simulink model "parallel_battery_SC_boost_converter_new"  (R2021a)
settings: Solver=ode23tb  StartTime=0.0  StopTime=20  RelTol=1e-3  EnableMultiTasking=on
undefined symbols (not defined in the file): Ion, Lithium, Ts
libraries: spsMosfetLib x9, spsSeriesRLCBranchLib x6, spsParallelRLCBranchLib x6, spsVoltageMeasurementLib x5, spsCurrentMeasurementLib x3, slpidlib x3, simulink x3, spsDiodeLib x2, spsThreePhaseParallelRLCLoadLib x1, spsBatteryLib x1, spsIGBTDiodeLib x1, spsThreePhaseVIMeasurementLib x1
settings Model: SimulationMode=accelerator  Creator=The MathWorks, Inc.  LastModifiedBy=JulianChung
settings SolverCC: AlgebraicLoopSolver=TrustRegion
settings DataIOCC: LimitDataPoints=on  SaveFormat=Array  ReturnWorkspaceOutputs=off
settings OptimizationCC: BlockReduction=off  DefaultParameterBehavior=Inlined  BufferReuse=off  ExpressionDepthLimit=2147483647  EfficientMapNaN2IntZero=off  LifeSpan=inf
settings DebuggingCC: UnderspecifiedInitializationDetection=Classic  MergeDetectMultiDrivingBlocksExec=none  SolverPrmCheckMsg=warning  FcnCallInpInsideContextMsg=warning  UnconnectedLineMsg=none  AllowSymbolicDim=off  StateNameClashWarn=warning  SFUnexpectedBacktrackingDiag=warning  SFNoUnconditionalDefaultTransitionDiag=warning  SFExecutionAtInitializationDiag=none  SFMachineParentedDataDiag=warning  ArithmeticOperatorsInVariantConditions=warning
settings HardwareCC: ProdBitPerPointer=32  ProdBitPerSizeT=32  ProdBitPerPtrDiffT=32  ProdLargestAtomicFloat=None  ProdIntDivRoundTo=Undefined  ProdEndianess=Unspecified  ProdWordSize=32  ProdHWDeviceType=32-bit Generic  TargetBitPerPointer=64  TargetBitPerSizeT=64  TargetBitPerPtrDiffT=64  TargetLongLongMode=on  TargetIntDivRoundTo=Zero  TargetEndianess=LittleEndian  TargetWordSize=64  TargetHWDeviceType=MATLAB Host  ProdEqTarget=off
settings ModelReferenceCC: PropagateSignalLabelsOutOfModel=off
settings SFSimCC: SimUseLocalCustomCode=off  CustomCodeUndefinedFunction=UseInterfaceOnly
settings RTWCC: SystemTargetFile=accel.tlc  TemplateMakefile=accel_default_tmf  RTWVerbose=off  RTWUseLocalCustomCode=off
settings CodeAppCC: MaxIdLength=128  StateflowObjectComments=on
settings STFCustomTargetCC: MATLABClassNameForMDSCustomization=Simulink.SoftwareTarget.TargetSpecificTriggerConfigurationBase  UseToolchainInfoCompliant=off  SystemTargetFile=accel.tlc
settings ConfigComp: CovMetricSettings=dw  CovSaveCumulativeToWorkspaceVar=on  CovSaveSingleToWorkspaceVar=on  CovExternalEMLEnable=off  CovSFcnEnable=off
settings SimscapeCC: SimscapeNormalizeSystem=off

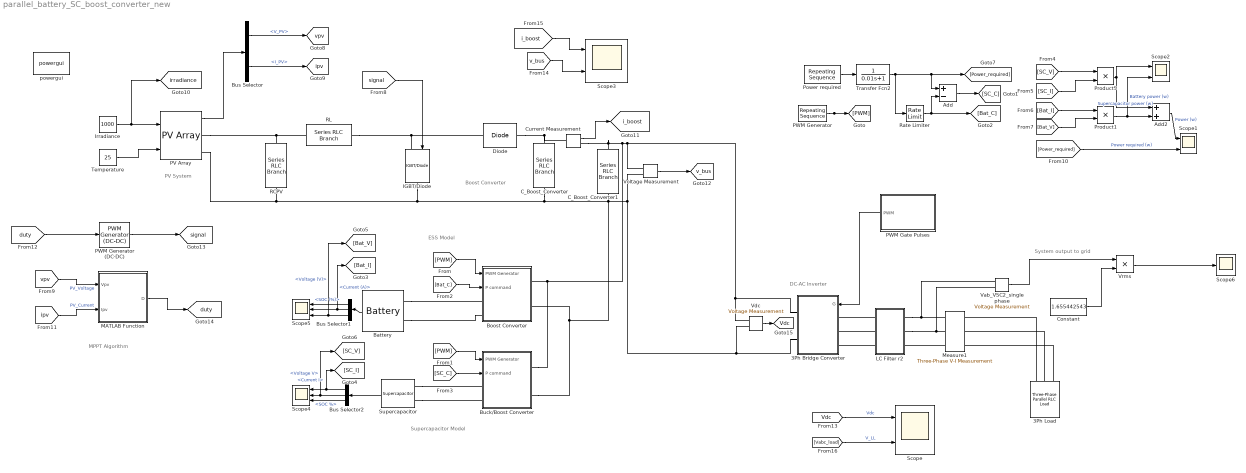
== system parallel_battery_SC_boost_converter_new ==
  note: Supercapacitor Model
  note: MPPT Algorithm
  note: PV System
  note: Boost Converter
  note: DC-AC Inverter
  note: System output to grid
  note: ESS Model
  "3Ph Load " : spsThreePhaseParallelRLCLoadLib/Three-Phase Parallel RLC Load  LConnTagsString=A|B|C  Configuration=Y (floating)  NominalVoltage=415  Vabc=[1e3 1e3 1e3]  Vabcp=[1e3 1e3 1e3]  NominalFrequency=50  UnbalancedPower=off  ActivePower=5e3  InductivePower=0  CapacitivePower=0  Pabc=[10e3 9e3 11e3]  QLabc=[100 90 110]  QCabc=[100 90 110]  Pabcp=[10e3 9e3 11e3]  QLabcp=[100 90 110]  QCabcp=[100 90 110]  Measurements=None  LoadType=constant Z
  3Ph Bridge Converter : Subsystem
  Add : Sum  Inputs=+-
  Add2 : Sum
  Battery : spsBatteryLib/Battery  BatType=Lithium-Ion  ShowTempParam=off  ThermalPreset=no  ShowAgeParam=off  NomV=26.4  NomQ=6.6  SOC=100  Batt_Tr=30  PresetModel=on  MaxQ=6.6  MinV=19.8  FullV=30.7293  Dis_rate=2.8696  R=0.04  Normal_OP=5.9687  expZone="[28.5222     0.324261]"  current=[6.5 13 32.5]  Units=Time  Tci=20  NomT=25  T2=0  MaxQ2=2.208  FullV2=3.45  Normal_OP2=2.8  expZone2="[3.22        0.23]"  Rca=0.6  ti=1000  Dp=0  Neq0=0  Tsim=1e6  Ta1=25  Qeol=5.4*0.9  Reol=0.013333*1.2  Char_age=[2.3478, 3]  Dis_age=[2.3478, 10]  N1=1500  N2=10500  N3=1000  N4=1400  Ta2=45  N5=950
  Boost Converter : Subsystem
  Buck/Boost Converter : Subsystem
  Bus Selector : BusSelector  OutputSignals=V_PV,I_PV
  Bus Selector1 : BusSelector  OutputSignals=SOC (%),Current (A),Voltage (V)
  Bus Selector2 : BusSelector  OutputSignals=Current I,Voltage V,SOC %
  C_Boost_Converter : spsSeriesRLCBranchLib/Series RLC Branch  LConnTagsString=__new0  RConnTagsString=__new0  BranchType=RC  Resistance=1e-4  Inductance=1e-3  SetiL0=off  InitialCurrent=0  Capacitance=3300e-6  Setx0=off  InitialVoltage=0  Measurements=None
  C_Boost_Converter1 : spsSeriesRLCBranchLib/Series RLC Branch  LConnTagsString=__new0  RConnTagsString=__new0  BranchType=R  Resistance=12  Inductance=1e-3  SetiL0=off  InitialCurrent=0  Capacitance=3300e-6  Setx0=off  InitialVoltage=0  Measurements=None
  Constant : Constant  Value=1.655442543
  Current Measurement : spsCurrentMeasurementLib/Current Measurement  PhasorSimulation=off  OutputType=Complex  PSBequivalent=0
  Diode : spsDiodeLib/Diode  Ron=0.001  Lon=0  Vf=0.8  IC=0  UseSnubber=0  Rs=500  Cs=250e-9  Measurements=off
  IGBT/Diode : spsIGBTDiodeLib/IGBT//Diode  Ron=1e-3  Rs=1e5  Cs=inf  Measurements=off
  Irradiance : Constant  Value=1000
  LC Filter r2 : Subsystem  mask{L=10e-3, C=20e-6}
      mask prompts: L "Inductance"; C "Capacitance"
  MATLAB Function : MATLAB Function  TreatAsAtomicUnit=on
  Measure1 : spsThreePhaseVIMeasurementLib/Three-Phase V-I Measurement  VoltageMeasurement=phase-to-phase  SetLabelV=on  LabelV=Vabc_load  Vpu=off  VpuLL=off  CurrentMeasurement=no  SetLabelI=off  LabelI=I1  Ipu=off  Pbase=1e3  Vbase=380  OutputType=Magnitude  PhasorSimulation=off  PSBequivalent=0
  PV Array : spsPVArrayLib/PV Array  Npar=10  Nser=3  PlotType=array @ 1000 W/m2 & specified temperatures  S_vec="[ 1000  500  100 ]"  Temp_C_vec="[ 45 25  ]"  ModuleName=User-defined  PlotWhenSelected=off  Pm=30  Ncell=20  Voc=12  Isc=4  Vm=10  Im=3  beta_Voc_pc=-0.318  alpha_Isc_pc=0.011  beta_Voc=-0.03816  alpha_Isc=0.00044  IL=4.052  I0=2.3913e-11  nI=0.9143  Rsh=11.0082  Rs=0.14305  RobustModel=off  RobustCellTemperature=313.3991  BAL=on  Tc=1e-6  Tfilter=5e-5
  PWM Gate Pulses : Subsystem  mask{fc=50, fs=20000, m=1, inj=off, shift=0}
      mask prompts: fc "Control signal freq(Fc)"; fs "Swicting frequency"; m "Modulation Index"; inj "3rd harmonic Injection"; shift "Phase shift(Degrees)"
  PWM Generator : simulink/Sources/Repeating Sequence  rep_seq_t="[0 1/4*0.0001  2/4*0.0001  3/4*0.0001  0.0001]"  rep_seq_y=[0 1 0 -1 0]
  PWM Generator (DC-DC) : spsPWMGeneratorDCDCLib/PWM Generator (DC-DC)  Fsw=5000  Ts=10e-6
  Power required : simulink/Sources/Repeating Sequence  rep_seq_t=[0 1 2 3 5 6 7 8 9 10]  rep_seq_y=[2000 1500 1250 1000 1000 1000 500 0 0 0 ]
  Product1 : Product  RndMeth=Zero
  Product5 : Product  RndMeth=Zero
  RCPV : spsSeriesRLCBranchLib/Series RLC Branch  LConnTagsString=__new0  RConnTagsString=__new0  BranchType=RC  Resistance=1e-4  Inductance=1e-3  SetiL0=off  InitialCurrent=0  Capacitance=100e-6  Setx0=off  InitialVoltage=0  Measurements=None
  RL : spsSeriesRLCBranchLib/Series RLC Branch  LConnTagsString=__new0  RConnTagsString=__new0  BranchType=RL  Resistance=0.1  Inductance=5e-3  SetiL0=off  InitialCurrent=0  Capacitance=100e-6  Setx0=off  InitialVoltage=0  Measurements=None
  Rate Limiter : RateLimiter  RisingSlewLimit=300  FallingSlewLimit=-300  SampleTimeMode=inherited
  Scope{,1..3} (4 alike) : Scope  NumInputPorts=2
  Scope4 : Scope  NumInputPorts=3
  Scope5 : Scope  NumInputPorts=3
  Scope6 : Scope
  Supercapacitor : spsSupercapacitorLib/Supercapacitor  C=500  Rdc=2.1e-3  Voltage=16  Ns=6  Np=1  Vinit=16  Temp=25  PresetModel=on  EstParam=off  Nc=1  r=1e-9  epsilon=6.0208e-10  Ich=10  Vstern="[0.161  2.7  7.8]"  Self_dis=on  Ioc=10  Vself="[48  47.8  47.06  44.65]"  demandeplot=off  I=10.2  Units=sec  Vmax=17  If=5.2e-3  deltaV=0.3  alpha=0.3  sec=1988
      settings: SourceProductBaseCode=PS
  Temperature : Constant  Value=25
  Transfer Fcn2 : TransferFcn  Denominator=[0.01 1]
  Vab_VSC2_single phase : spsVoltageMeasurementLib/Voltage Measurement  Tag=PoWeRsYsTeMmEaSuReMeNt  PhasorSimulation=off  OutputType=Magnitude  PSBequivalent=0
  "Vdc " : spsVoltageMeasurementLib/Voltage Measurement  Tag=PoWeRsYsTeMmEaSuReMeNt  PhasorSimulation=off  OutputType=Magnitude  PSBequivalent=0
  Voltage Measurement : spsVoltageMeasurementLib/Voltage Measurement  PhasorSimulation=off  OutputType=Complex  PSBequivalent=0
  Vrms : Product
  powergui : spspowerguiLib/powergui  Priority=1  SimulationMode=Discrete  SampleTime=10e-6  frequency=60  Iterations=50  frequencyindice=0  Pbase=100e6  ErrMax=1e-4  UnitsV=kV  UnitsW=MW  buscounter=0  FunctionMessages=off  echomessages=off  EnableUseOfTLC=off  CurrentSourceSwitches=off  DisableSnubberDevices=off  DisableRonSwitches=off  DisableVfSwitches=off  DisplayEquations=off  AutomaticDiscreteSolvers=off  SolverType=Tustin/Backward Euler (TBE)  Interpol=off  ExternalGateDelay=off  methode=off  Ts=0  x0status=blocks  SPID=off  SwTol=0  HookPort=off  NonlinearTolerance=1e-4  nMaxIteration=100  ContinueOnMaxIteration=off  RestoreLinks=warning  ResistiveCurrentMeasurement=off  Frange=[0:1:1000]  Ylog=on  Xlog=on  ShowGrid=on  save=on  variable=ZDa  structure=donnee  ZoomFFT=off  StartTime=0.0  cycles=1  DisplayStyle=1  fundamental=60  FreqAxis=off  MaxFrequency=1000  frequencyindicesteady=10  RmsSteady=1  display=off
  tag scope: Vdc=global, duty=global, i_boost=global, ipv=global, irradiance=global, signal=global, v_bus=global, vpv=global
  wires:
  Battery/1 -> Bus Selector1/1
  Bus Selector1/1 -> Scope5/1  "<SOC (%)>"
  Bus Selector1/2 -> [Bat_I], Scope5/2  "<Current (A)>"
  Bus Selector1/3 -> Scope5/3, [Bat_V]  "<Voltage (V)>"
  Transfer Fcn2/1 -> Rate Limiter/1, Add/1, [Power_required]
  Rate Limiter/1 -> Add/2, [Bat_C]
  Power required/1 -> Transfer Fcn2/1
  PWM Generator/1 -> [PWM]
  [PWM] -> Boost Converter/1(PWM Generator)
  [Bat_C] -> Boost Converter/2(P command)
  [PWM] -> Buck/Boost Converter/1(PWM Generator)
  [SC_C] -> Buck/Boost Converter/2(P command)
  Add/1 -> [SC_C]
  Bus Selector2/1 -> [SC_I], Scope4/1  "<Current I>"
  Bus Selector2/2 -> Scope4/2, [SC_V]  "<Voltage V>"
  Bus Selector2/3 -> Scope4/3  "<SOC %>"
  Supercapacitor/1 -> Bus Selector2/1
  [Bat_I] -> Product1/1
  [Bat_V] -> Product1/2
  [SC_V] -> Product5/1
  [SC_I] -> Product5/2
  Product5/1 -> Add2/1, Scope2/1  "Supercapacitor power (w)"
  Product1/1 -> Add2/2, Scope2/2  "Battery power (w)"
  [Power_required] -> Scope1/2  "Power required (w)"
  Add2/1 -> Scope1/1  "Power (w)"
  Bus Selector/1 -> [vpv]  "<V_PV>"
  Voltage Measurement/1 -> [v_bus]
  Current Measurement/1 -> [i_boost]
  [signal] -> IGBT/Diode/1
  PV Array/1 -> Bus Selector/1
  Bus Selector/2 -> [ipv]  "<I_PV>"
  Irradiance/1 -> [irradiance], PV Array/1
  Temperature/1 -> PV Array/2
  [ipv] -> MATLAB Function/2(Ipv)  "PV_Current"
  [vpv] -> MATLAB Function/1(Vpv)  "PV_Voltage"
  MATLAB Function/1(D) -> [duty]
  PWM Generator (DC-DC)/1 -> [signal]
  [duty] -> PWM Generator (DC-DC)/1
  [i_boost] -> Scope3/1
  [v_bus] -> Scope3/2
  PWM Gate Pulses/1(PWM) -> 3Ph Bridge Converter/1(G)
  "Vdc "/1 -> [Vdc]
  [Vdc] -> Scope/1  "Vdc"
  [Vabc_load] -> Scope/2  "V_LL"
  Vab_VSC2_single phase/1 -> Vrms/1
  Constant/1 -> Vrms/2
  Vrms/1 -> Scope6/1
  connections:
  Supercapacitor/LConn1 -- Buck/Boost Converter/LConn1
  Supercapacitor/LConn2 -- Buck/Boost Converter/LConn2
  Battery/LConn1 -- Boost Converter/LConn1
  Battery/LConn2 -- Boost Converter/LConn2
  3Ph Bridge Converter/RConn2 -- "Vdc "/LConn2 -- Voltage Measurement/LConn2 -- Boost Converter/RConn2 -- Buck/Boost Converter/RConn2 -- C_Boost_Converter1/RConn1 -- RCPV/RConn1 -- PV Array/RConn2 -- IGBT/Diode/RConn1 -- C_Boost_Converter/RConn1
  Diode/LConn1 -- RL/LConn1 -- IGBT/Diode/LConn1
  3Ph Bridge Converter/RConn1 -- C_Boost_Converter1/LConn1 -- Current Measurement/RConn1 -- Boost Converter/RConn1 -- Buck/Boost Converter/RConn1 -- Voltage Measurement/LConn1 -- "Vdc "/LConn1
  RCPV/LConn1 -- RL/RConn1 -- PV Array/RConn1
  Diode/RConn1 -- C_Boost_Converter/LConn1 -- Current Measurement/LConn1
  Measure1/LConn2 -- Vab_VSC2_single phase/LConn2 -- LC Filter r2/RConn2
  LC Filter r2/RConn1 -- Vab_VSC2_single phase/LConn1 -- Measure1/LConn1
  Measure1/LConn3 -- LC Filter r2/RConn3
  "3Ph Load "/LConn1 -- Measure1/RConn1
  LC Filter r2/LConn2 -- 3Ph Bridge Converter/LConn2
  "3Ph Load "/LConn2 -- Measure1/RConn2
  LC Filter r2/LConn3 -- 3Ph Bridge Converter/LConn3
  LC Filter r2/LConn1 -- 3Ph Bridge Converter/LConn1
  "3Ph Load "/LConn3 -- Measure1/RConn3

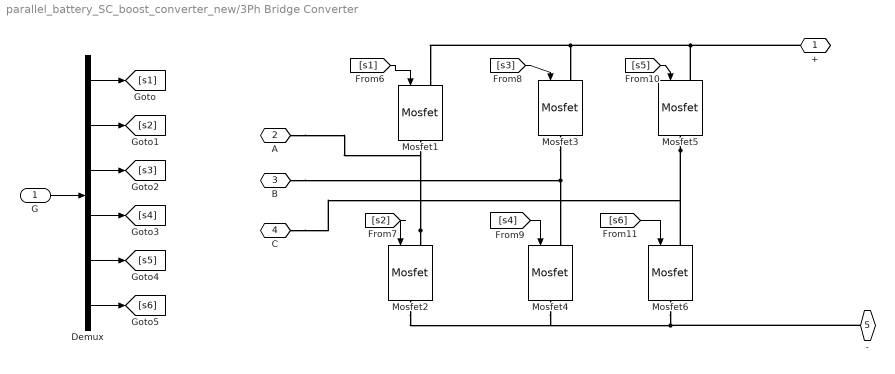
== system parallel_battery_SC_boost_converter_new/3Ph Bridge Converter ==
  G : Inport
  Demux : Demux  Outputs=6
  Mosfet{1..6} (6 alike) : spsMosfetLib/Mosfet  Ron=0.1  Lon=0  Rd=0.01  Vfd=0  IC=0  Rs=1e5  Cs=inf  Measurements=off
  + : PMIOPort  Side=Right
  A : PMIOPort  Port=2  Side=Left
  B : PMIOPort  Port=3  Side=Left
  C : PMIOPort  Port=4  Side=Left
  - : PMIOPort  Port=5  Side=Right
  wires:
  [s1] -> Mosfet1/1
  [s2] -> Mosfet2/1
  [s3] -> Mosfet3/1
  [s4] -> Mosfet4/1
  [s5] -> Mosfet5/1
  [s6] -> Mosfet6/1
  Demux/1 -> [s1]
  Demux/2 -> [s2]
  Demux/3 -> [s3]
  Demux/4 -> [s4]
  Demux/5 -> [s5]
  Demux/6 -> [s6]
  G/1 -> Demux/1
  connections:
  Mosfet5/LConn1 -- Mosfet1/LConn1 -- Mosfet3/LConn1 -- +/RConn1
  Mosfet6/RConn1 -- Mosfet2/RConn1 -- Mosfet4/RConn1 -- -/RConn1
  Mosfet2/LConn1 -- Mosfet1/RConn1 -- A/RConn1
  Mosfet3/RConn1 -- Mosfet4/LConn1 -- B/RConn1
  Mosfet5/RConn1 -- Mosfet6/LConn1 -- C/RConn1

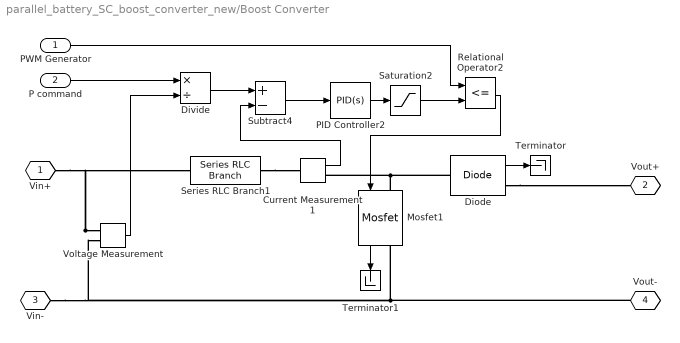
== system parallel_battery_SC_boost_converter_new/Boost Converter ==
  PWM Generator : Inport
  P command : Inport  Port=2
  Current Measurement1 : spsCurrentMeasurementLib/Current Measurement  PhasorSimulation=off  OutputType=Complex  PSBequivalent=0
  Diode : spsDiodeLib/Diode  Ron=0.001  Lon=0  Vf=0.8  IC=0  UseSnubber=off  Rs=500  Cs=250e-9  Measurements=on
  Divide : Product  Inputs=*/
  Mosfet1 : spsMosfetLib/Mosfet  Ron=0.1  Lon=0  Rd=0.01  Vfd=0  IC=0  Rs=1e5  Cs=inf  Measurements=on
  PID Controller2 : slpidlib/PID Controller  Controller=PID  Form=Parallel  TimeDomain=Continuous-time  UseExternalTs=off  SampleTime=-1  IntegratorMethod=Forward Euler  FilterMethod=Forward Euler  ControllerParametersSource=internal  P=1.5  I=1  D=0  UseFilter=on  N=100  TunerSelectOption=Transfer Function Based (PID Tuner App)  InitialConditionSource=internal  InitialConditionForIntegrator=0  InitialConditionForFilter=0  DifferentiatorICPrevScaledInput=0  ExternalReset=none  TrackingMode=off  Kt=1  LimitOutput=off  SatLimitsSource=internal  UpperSaturationLimit=inf  LowerSaturationLimit=-inf  LinearizeAsGain=off  AntiWindupMode=none  Kb=1  POutMin=[]  POutMax=[]  IOutMin=[]  IOutMax=[]  DOutMin=[]  DOutMax=[]  NOutMin=[]  NOutMax=[]  SumOutMin=[]  SumOutMax=[]  SaturationOutMin=[]  SaturationOutMax=[]  PParamMin=[]  PParamMax=[]  IParamMin=[]  IParamMax=[]  DParamMin=[]  DParamMax=[]  NParamMin=[]  NParamMax=[]  KbParamMin=[]  KbParamMax=[]  KtParamMin=[]  KtParamMax=[]  KbOutMin=[]  KbOutMax=[]  KtOutMin=[]  KtOutMax=[]  IntegratorOutMin=[]  IntegratorOutMax=[]  FilterOutMin=[]  FilterOutMax=[]  SumI1OutMin=[]  SumI1OutMax=[]  SumI2OutMin=[]  SumI2OutMax=[]  SumI3OutMin=[]  SumI3OutMax=[]  SumI4OutMin=[]  SumI4OutMax=[]  SumDOutMin=[]  SumDOutMax=[]  DifferentiatorOutMin=[]  DifferentiatorOutMax=[]  FilterDiffOutCoefMin=[]  FilterDiffOutCoefMax=[]  ReciprocalOutMin=[]  ReciprocalOutMax=[]  SumDenOutMin=[]  SumDenOutMax=[]  SumNumOutMin=[]  SumNumOutMax=[]  DivideOutMin=[]  DivideOutMax=[]  UdiffTsProdOutMin=[]  UdiffTsProdOutMax=[]  NTsProdOutMin=[]  NTsProdOutMax=[]  UintegralTsProdOutMin=[]  UintegralTsProdOutMax=[]  UngainTsProdOutMin=[]  UngainTsProdOutMax=[]  IntegratorContinuousStateAttributes=''  IntegratorStateMustResolveToSignalObject=off  IntegratorRTWStateStorageClass=Auto  FilterContinuousStateAttributes=''  FilterStateMustResolveToSignalObject=off  FilterRTWStateStorageClass=Auto  ParallelPVariant=InternalParameters  IdealPVariant=Disabled  IVariant=InternalParameters  DVariant=InternalParameters  IntegratorVariant=Continuous  SatVariant=Disabled  AWVariant=Passthrough  PCopyVariant=Disabled  TRVariant=Disabled  FdbkBlocksVariant=Forward  IdealPFdbkVariant=Disabled  SatFdbkVariant=Disabled  DerivativeFilterVariant=ContFilter  NVariant=InternalParameters  NCopyVariant=Disabled  FilterICVariant=InternalICsFilter  IntegratorICVariant=InternalICs  ExternalResetVariant=Disabled  TRSumVariant=Passthrough  SumFdbkVariant=Disabled  SumVariant=Sum_PID  TsampFilterVariant=InternalTs  TsampNgainVariant=Passthrough  TsampIntegralVariant=Passthrough  ExternalSaturationOutDataTypeStr=Inherit: Same as second input
  Relational Operator2 : RelationalOperator  Operator=<=  OutDataTypeStr=boolean  RndMeth=Nearest
  Saturation2 : Saturate  UpperLimit=1  LowerLimit=-1
  Series RLC Branch1 : spsSeriesRLCBranchLib/Series RLC Branch  LConnTagsString=__new0  RConnTagsString=__new0  BranchType=L  Resistance=1  Inductance=1e-3  SetiL0=off  InitialCurrent=0  Capacitance=1e-6  Setx0=off  InitialVoltage=0  Measurements=None
  Subtract4 : Sum  Inputs=+-
  Terminator : Terminator
  Terminator1 : Terminator
  Voltage Measurement : spsVoltageMeasurementLib/Voltage Measurement  PhasorSimulation=off  OutputType=Complex  PSBequivalent=0
  Vin+ : PMIOPort  Tag=PMCPort  Side=Left
  Vout+ : PMIOPort  Tag=PMCPort  Port=2  Side=Right
  Vin- : PMIOPort  Tag=PMCPort  Port=3  Side=Left
  Vout- : PMIOPort  Tag=PMCPort  Port=4  Side=Right
  wires:
  Voltage Measurement/1 -> Divide/2
  P command/1 -> Divide/1
  Divide/1 -> Subtract4/1
  Relational Operator2/1 -> Mosfet1/1
  Current Measurement1/1 -> Subtract4/2
  PWM Generator/1 -> Relational Operator2/1
  Subtract4/1 -> PID Controller2/1
  PID Controller2/1 -> Saturation2/1
  Saturation2/1 -> Relational Operator2/2
  Diode/1 -> Terminator/1
  Mosfet1/1 -> Terminator1/1
  connections:
  Series RLC Branch1/RConn1 -- Current Measurement1/LConn1
  Vout-/RConn1 -- Voltage Measurement/LConn2 -- Vin-/RConn1 -- Mosfet1/RConn1
  Voltage Measurement/LConn1 -- Series RLC Branch1/LConn1 -- Vin+/RConn1
  Diode/LConn1 -- Current Measurement1/RConn1 -- Mosfet1/LConn1
  Diode/RConn1 -- Vout+/RConn1

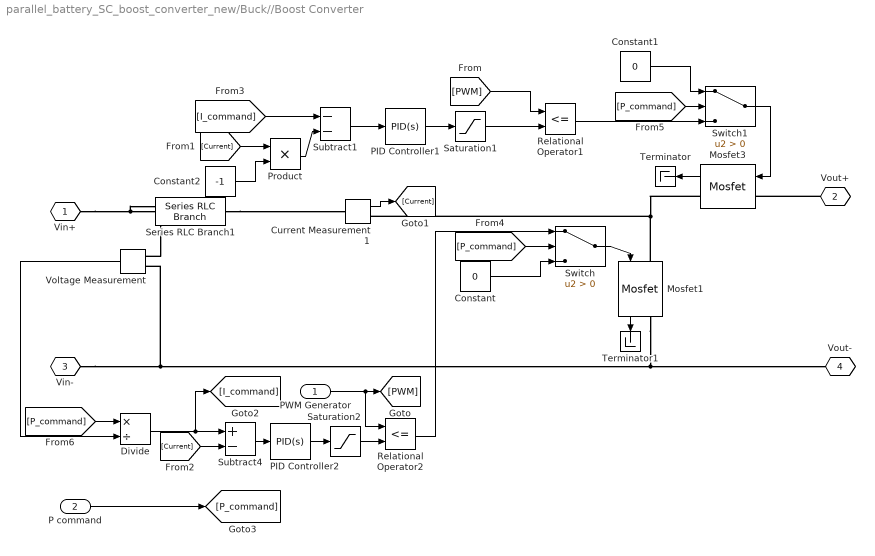
== system parallel_battery_SC_boost_converter_new/Buck//Boost Converter ==
  PWM Generator : Inport
  P command : Inport  Port=2
  Constant : Constant  Value=0
  Constant1 : Constant  Value=0
  Constant2 : Constant  Value=-1
  Current Measurement1 : spsCurrentMeasurementLib/Current Measurement  PhasorSimulation=off  OutputType=Complex  PSBequivalent=0
  Divide : Product  Inputs=*/
  Mosfet1 : spsMosfetLib/Mosfet  Ron=0.1  Lon=0  Rd=0.01  Vfd=0  IC=0  Rs=1e5  Cs=inf  Measurements=on
  Mosfet3 : spsMosfetLib/Mosfet  Ron=0.1  Lon=0  Rd=0.01  Vfd=0  IC=0  Rs=1e5  Cs=inf  Measurements=on
  PID Controller1 : slpidlib/PID Controller  Controller=PID  Form=Parallel  TimeDomain=Continuous-time  UseExternalTs=off  SampleTime=-1  IntegratorMethod=Forward Euler  FilterMethod=Forward Euler  ControllerParametersSource=internal  P=1.5  I=1  D=0  UseFilter=on  N=100  TunerSelectOption=Transfer Function Based (PID Tuner App)  InitialConditionSource=internal  InitialConditionForIntegrator=0  InitialConditionForFilter=0  DifferentiatorICPrevScaledInput=0  ExternalReset=none  TrackingMode=off  Kt=1  LimitOutput=off  SatLimitsSource=internal  UpperSaturationLimit=inf  LowerSaturationLimit=-inf  LinearizeAsGain=off  AntiWindupMode=none  Kb=1  POutMin=[]  POutMax=[]  IOutMin=[]  IOutMax=[]  DOutMin=[]  DOutMax=[]  NOutMin=[]  NOutMax=[]  SumOutMin=[]  SumOutMax=[]  SaturationOutMin=[]  SaturationOutMax=[]  PParamMin=[]  PParamMax=[]  IParamMin=[]  IParamMax=[]  DParamMin=[]  DParamMax=[]  NParamMin=[]  NParamMax=[]  KbParamMin=[]  KbParamMax=[]  KtParamMin=[]  KtParamMax=[]  KbOutMin=[]  KbOutMax=[]  KtOutMin=[]  KtOutMax=[]  IntegratorOutMin=[]  IntegratorOutMax=[]  FilterOutMin=[]  FilterOutMax=[]  SumI1OutMin=[]  SumI1OutMax=[]  SumI2OutMin=[]  SumI2OutMax=[]  SumI3OutMin=[]  SumI3OutMax=[]  SumI4OutMin=[]  SumI4OutMax=[]  SumDOutMin=[]  SumDOutMax=[]  DifferentiatorOutMin=[]  DifferentiatorOutMax=[]  FilterDiffOutCoefMin=[]  FilterDiffOutCoefMax=[]  ReciprocalOutMin=[]  ReciprocalOutMax=[]  SumDenOutMin=[]  SumDenOutMax=[]  SumNumOutMin=[]  SumNumOutMax=[]  DivideOutMin=[]  DivideOutMax=[]  UdiffTsProdOutMin=[]  UdiffTsProdOutMax=[]  NTsProdOutMin=[]  NTsProdOutMax=[]  UintegralTsProdOutMin=[]  UintegralTsProdOutMax=[]  UngainTsProdOutMin=[]  UngainTsProdOutMax=[]  IntegratorContinuousStateAttributes=''  IntegratorStateMustResolveToSignalObject=off  IntegratorRTWStateStorageClass=Auto  FilterContinuousStateAttributes=''  FilterStateMustResolveToSignalObject=off  FilterRTWStateStorageClass=Auto  ParallelPVariant=InternalParameters  IdealPVariant=Disabled  IVariant=InternalParameters  DVariant=InternalParameters  IntegratorVariant=Continuous  SatVariant=Disabled  AWVariant=Passthrough  PCopyVariant=Disabled  TRVariant=Disabled  FdbkBlocksVariant=Forward  IdealPFdbkVariant=Disabled  SatFdbkVariant=Disabled  DerivativeFilterVariant=ContFilter  NVariant=InternalParameters  NCopyVariant=Disabled  FilterICVariant=InternalICsFilter  IntegratorICVariant=InternalICs  ExternalResetVariant=Disabled  TRSumVariant=Passthrough  SumFdbkVariant=Disabled  SumVariant=Sum_PID  TsampFilterVariant=InternalTs  TsampNgainVariant=Passthrough  TsampIntegralVariant=Passthrough  ExternalSaturationOutDataTypeStr=Inherit: Same as second input
  PID Controller2 : slpidlib/PID Controller  Controller=PID  Form=Parallel  TimeDomain=Continuous-time  UseExternalTs=off  SampleTime=-1  IntegratorMethod=Forward Euler  FilterMethod=Forward Euler  ControllerParametersSource=internal  P=1.5  I=1  D=0  UseFilter=on  N=100  TunerSelectOption=Transfer Function Based (PID Tuner App)  InitialConditionSource=internal  InitialConditionForIntegrator=0  InitialConditionForFilter=0  DifferentiatorICPrevScaledInput=0  ExternalReset=none  TrackingMode=off  Kt=1  LimitOutput=off  SatLimitsSource=internal  UpperSaturationLimit=inf  LowerSaturationLimit=-inf  LinearizeAsGain=off  AntiWindupMode=none  Kb=1  POutMin=[]  POutMax=[]  IOutMin=[]  IOutMax=[]  DOutMin=[]  DOutMax=[]  NOutMin=[]  NOutMax=[]  SumOutMin=[]  SumOutMax=[]  SaturationOutMin=[]  SaturationOutMax=[]  PParamMin=[]  PParamMax=[]  IParamMin=[]  IParamMax=[]  DParamMin=[]  DParamMax=[]  NParamMin=[]  NParamMax=[]  KbParamMin=[]  KbParamMax=[]  KtParamMin=[]  KtParamMax=[]  KbOutMin=[]  KbOutMax=[]  KtOutMin=[]  KtOutMax=[]  IntegratorOutMin=[]  IntegratorOutMax=[]  FilterOutMin=[]  FilterOutMax=[]  SumI1OutMin=[]  SumI1OutMax=[]  SumI2OutMin=[]  SumI2OutMax=[]  SumI3OutMin=[]  SumI3OutMax=[]  SumI4OutMin=[]  SumI4OutMax=[]  SumDOutMin=[]  SumDOutMax=[]  DifferentiatorOutMin=[]  DifferentiatorOutMax=[]  FilterDiffOutCoefMin=[]  FilterDiffOutCoefMax=[]  ReciprocalOutMin=[]  ReciprocalOutMax=[]  SumDenOutMin=[]  SumDenOutMax=[]  SumNumOutMin=[]  SumNumOutMax=[]  DivideOutMin=[]  DivideOutMax=[]  UdiffTsProdOutMin=[]  UdiffTsProdOutMax=[]  NTsProdOutMin=[]  NTsProdOutMax=[]  UintegralTsProdOutMin=[]  UintegralTsProdOutMax=[]  UngainTsProdOutMin=[]  UngainTsProdOutMax=[]  IntegratorContinuousStateAttributes=''  IntegratorStateMustResolveToSignalObject=off  IntegratorRTWStateStorageClass=Auto  FilterContinuousStateAttributes=''  FilterStateMustResolveToSignalObject=off  FilterRTWStateStorageClass=Auto  ParallelPVariant=InternalParameters  IdealPVariant=Disabled  IVariant=InternalParameters  DVariant=InternalParameters  IntegratorVariant=Continuous  SatVariant=Disabled  AWVariant=Passthrough  PCopyVariant=Disabled  TRVariant=Disabled  FdbkBlocksVariant=Forward  IdealPFdbkVariant=Disabled  SatFdbkVariant=Disabled  DerivativeFilterVariant=ContFilter  NVariant=InternalParameters  NCopyVariant=Disabled  FilterICVariant=InternalICsFilter  IntegratorICVariant=InternalICs  ExternalResetVariant=Disabled  TRSumVariant=Passthrough  SumFdbkVariant=Disabled  SumVariant=Sum_PID  TsampFilterVariant=InternalTs  TsampNgainVariant=Passthrough  TsampIntegralVariant=Passthrough  ExternalSaturationOutDataTypeStr=Inherit: Same as second input
  Product : Product  RndMeth=Zero
  Relational Operator1 : RelationalOperator  Operator=<=  OutDataTypeStr=boolean  RndMeth=Nearest
  Relational Operator2 : RelationalOperator  Operator=<=  OutDataTypeStr=boolean  RndMeth=Nearest
  Saturation1 : Saturate  UpperLimit=1  LowerLimit=-1
  Saturation2 : Saturate  UpperLimit=1  LowerLimit=-1
  Series RLC Branch1 : spsSeriesRLCBranchLib/Series RLC Branch  LConnTagsString=__new0  RConnTagsString=__new0  BranchType=L  Resistance=1  Inductance=1e-3  SetiL0=off  InitialCurrent=0  Capacitance=1e-6  Setx0=off  InitialVoltage=0  Measurements=None
  Subtract1 : Sum  Inputs=--
  Subtract4 : Sum  Inputs=+-
  Switch : Switch  Criteria=u2 > Threshold
  Switch1 : Switch  Criteria=u2 > Threshold
  Terminator : Terminator
  Terminator1 : Terminator
  Voltage Measurement : spsVoltageMeasurementLib/Voltage Measurement  PhasorSimulation=off  OutputType=Complex  PSBequivalent=0
  Vin+ : PMIOPort  Tag=PMCPort  Side=Left
  Vout+ : PMIOPort  Tag=PMCPort  Port=2  Side=Right
  Vin- : PMIOPort  Tag=PMCPort  Port=3  Side=Left
  Vout- : PMIOPort  Tag=PMCPort  Port=4  Side=Right
  wires:
  Saturation2/1 -> Relational Operator2/2
  PID Controller2/1 -> Saturation2/1
  Subtract4/1 -> PID Controller2/1
  PWM Generator/1 -> Relational Operator2/1, [PWM]
  Divide/1 -> [I_command], Subtract4/1
  P command/1 -> [P_command]
  Switch/1 -> Mosfet1/1
  Saturation1/1 -> Relational Operator1/2
  PID Controller1/1 -> Saturation1/1
  Subtract1/1 -> PID Controller1/1
  [PWM] -> Relational Operator1/1
  [Current] -> Subtract4/2
  [Current] -> Product/1
  Product/1 -> Subtract1/2
  Constant2/1 -> Product/2
  [I_command] -> Subtract1/1
  Current Measurement1/1 -> [Current]
  Switch1/1 -> Mosfet3/1
  Relational Operator2/1 -> Switch/1
  Constant/1 -> Switch/3
  Constant1/1 -> Switch1/1
  Mosfet3/1 -> Terminator/1
  Mosfet1/1 -> Terminator1/1
  Relational Operator1/1 -> Switch1/3
  [P_command] -> Switch/2
  [P_command] -> Switch1/2
  [P_command] -> Divide/1
  Voltage Measurement/1 -> Divide/2
  connections:
  Vin-/RConn1 -- Voltage Measurement/LConn2 -- Vout-/RConn1 -- Mosfet1/RConn1
  Vin+/RConn1 -- Series RLC Branch1/LConn1 -- Voltage Measurement/LConn1
  Mosfet1/LConn1 -- Current Measurement1/RConn1 -- Mosfet3/RConn1
  Series RLC Branch1/RConn1 -- Current Measurement1/LConn1
  Vout+/RConn1 -- Mosfet3/LConn1

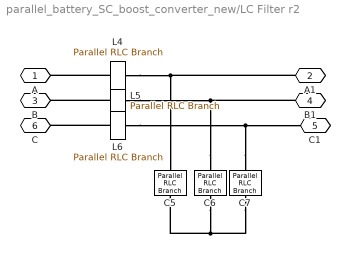
== system parallel_battery_SC_boost_converter_new/LC Filter r2 ==
  C5 : spsParallelRLCBranchLib/Parallel RLC Branch  LConnTagsString=a  RConnTagsString=__new0  BranchType=C  Resistance=inf  Inductance=inf  SetiL0=off  InitialCurrent=0  Capacitance=C  Setx0=off  InitialVoltage=0  Measurements=None
  C6 : spsParallelRLCBranchLib/Parallel RLC Branch  LConnTagsString=a  RConnTagsString=__new0  BranchType=C  Resistance=inf  Inductance=inf  SetiL0=off  InitialCurrent=0  Capacitance=C  Setx0=off  InitialVoltage=0  Measurements=None
  C7 : spsParallelRLCBranchLib/Parallel RLC Branch  LConnTagsString=a  RConnTagsString=__new0  BranchType=C  Resistance=inf  Inductance=inf  SetiL0=off  InitialCurrent=0  Capacitance=C  Setx0=off  InitialVoltage=0  Measurements=None
  L4 : spsParallelRLCBranchLib/Parallel RLC Branch  LConnTagsString=a  RConnTagsString=__new0  BranchType=L  Resistance=inf  Inductance=L  SetiL0=off  InitialCurrent=0  Capacitance=1.3e-3  Setx0=off  InitialVoltage=0  Measurements=None
  L5 : spsParallelRLCBranchLib/Parallel RLC Branch  LConnTagsString=a  RConnTagsString=__new0  BranchType=L  Resistance=inf  Inductance=L  SetiL0=off  InitialCurrent=0  Capacitance=1.3e-3  Setx0=off  InitialVoltage=0  Measurements=None
  L6 : spsParallelRLCBranchLib/Parallel RLC Branch  LConnTagsString=a  RConnTagsString=__new0  BranchType=L  Resistance=inf  Inductance=L  SetiL0=off  InitialCurrent=0  Capacitance=1.3e-3  Setx0=off  InitialVoltage=0  Measurements=None
  A : PMIOPort  Side=Left
  A1 : PMIOPort  Port=2  Side=Right
  B : PMIOPort  Port=3  Side=Left
  B1 : PMIOPort  Port=4  Side=Right
  C1 : PMIOPort  Port=5  Side=Right
  C : PMIOPort  Port=6  Side=Left
  connections:
  L4/LConn1 -- A/RConn1
  L6/LConn1 -- C/RConn1
  C5/RConn1 -- C7/RConn1 -- C6/RConn1
  L5/LConn1 -- B/RConn1
  C6/LConn1 -- B1/RConn1 -- L5/RConn1
  L4/RConn1 -- A1/RConn1 -- C5/LConn1
  C7/LConn1 -- C1/RConn1 -- L6/RConn1

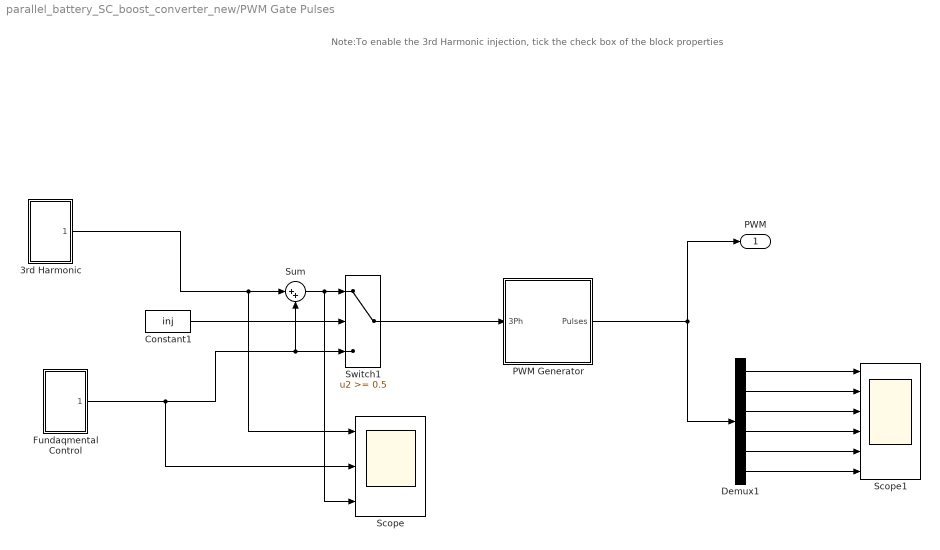
== system parallel_battery_SC_boost_converter_new/PWM Gate Pulses ==
  note: Note:To enable the 3rd Harmonic injection, tick the check box of the block properties
  3rd Harmonic : Subsystem
  Constant1 : Constant  Value=inj  SampleTime=Ts
  Demux1 : Demux  Outputs=6
  Fundaqmental Control : Subsystem
  PWM Generator : Subsystem  InitFcn=Ts=2e-6
  Scope : Scope  NumInputPorts=3
  Scope1 : Scope  NumInputPorts=6
  Sum : Sum  Inputs=|++
  Switch1 : Switch  Threshold=0.5  SampleTime=Ts  SaturateOnIntegerOverflow=on  InputSameDT=on
  PWM : Outport
  wires:
  Demux1/1 -> Scope1/1
  Demux1/2 -> Scope1/2
  Demux1/3 -> Scope1/3
  Demux1/4 -> Scope1/4
  Demux1/5 -> Scope1/5
  Demux1/6 -> Scope1/6
  PWM Generator/1(Pulses) -> PWM/1, Demux1/1
  Constant1/1 -> Switch1/2
  Switch1/1 -> PWM Generator/1(3Ph)
  Sum/1 -> Scope/3, Switch1/1
  3rd Harmonic/1(Sin(3wt)) -> Scope/1, Sum/1
  Fundaqmental Control/1(Sin(wt)) -> Scope/2, Sum/2, Switch1/3

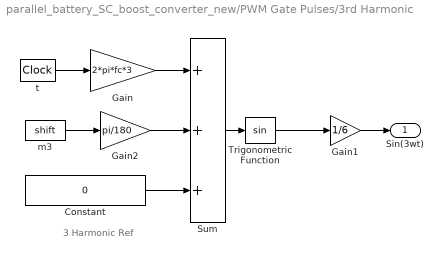
== system parallel_battery_SC_boost_converter_new/PWM Gate Pulses/3rd Harmonic ==
  note: 3 Harmonic Ref
  Constant : Constant  Value=0  SampleTime=Ts
  Gain : Gain  Gain=2*pi*fc*3  SaturateOnIntegerOverflow=on  OutDataTypeStr=Inherit: Same as input  ParamDataTypeStr=Inherit: Same as input
  Gain1 : Gain  Gain=1/6
  Gain2 : Gain  Gain=pi/180  SaturateOnIntegerOverflow=on  OutDataTypeStr=Inherit: Same as input  ParamDataTypeStr=Inherit: Same as input
  Sum : Sum  Inputs=+++  InputSameDT=on  SaturateOnIntegerOverflow=on  SampleTime=Ts  OutDataTypeStr=Inherit: Same as first input
  Trigonometric Function : Trigonometry  SampleTime=Ts
  m3 : Constant  Value=shift  SampleTime=Ts
  t : DigitalClock  SampleTime=Ts
  Sin(3wt) : Outport
  wires:
  t/1 -> Gain/1
  Gain/1 -> Sum/1
  Gain2/1 -> Sum/2
  m3/1 -> Gain2/1
  Constant/1 -> Sum/3
  Sum/1 -> Trigonometric Function/1
  Trigonometric Function/1 -> Gain1/1
  Gain1/1 -> Sin(3wt)/1

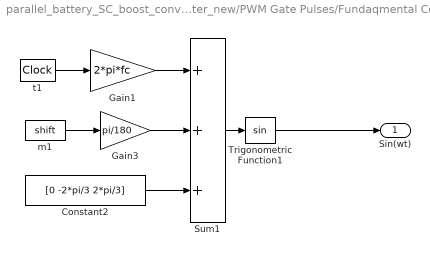
== system parallel_battery_SC_boost_converter_new/PWM Gate Pulses/Fundaqmental Control ==
  Constant2 : Constant  Value=[0 -2*pi/3 2*pi/3]  SampleTime=Ts
  Gain1 : Gain  Gain=2*pi*fc  SaturateOnIntegerOverflow=on  OutDataTypeStr=Inherit: Same as input  ParamDataTypeStr=Inherit: Same as input
  Gain3 : Gain  Gain=pi/180  SaturateOnIntegerOverflow=on  OutDataTypeStr=Inherit: Same as input  ParamDataTypeStr=Inherit: Same as input
  Sum1 : Sum  Inputs=+++  InputSameDT=on  SaturateOnIntegerOverflow=on  SampleTime=Ts  OutDataTypeStr=Inherit: Same as first input
  Trigonometric Function1 : Trigonometry  SampleTime=Ts
  m1 : Constant  Value=shift  SampleTime=Ts
  t1 : DigitalClock  SampleTime=Ts
  Sin(wt) : Outport
  wires:
  Trigonometric Function1/1 -> Sin(wt)/1
  t1/1 -> Gain1/1
  Gain1/1 -> Sum1/1
  Gain3/1 -> Sum1/2
  m1/1 -> Gain3/1
  Constant2/1 -> Sum1/3
  Sum1/1 -> Trigonometric Function1/1

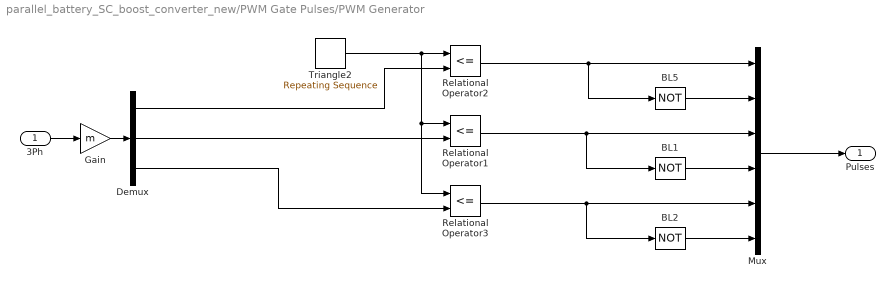
== system parallel_battery_SC_boost_converter_new/PWM Gate Pulses/PWM Generator ==
  3Ph : Inport
  BL1 : Logic  Operator=NOT  Inputs=1  SampleTime=Ts
  BL2 : Logic  Operator=NOT  Inputs=1  SampleTime=Ts
  BL5 : Logic  Operator=NOT  Inputs=1  SampleTime=Ts
  Demux : Demux  Outputs=3
  Gain : Gain  Gain=m
  Mux : Mux  Inputs=6
  Relational Operator1 : RelationalOperator  Operator=<=  RndMeth=Nearest
  Relational Operator2 : RelationalOperator  Operator=<=  RndMeth=Nearest
  Relational Operator3 : RelationalOperator  Operator=<=  RndMeth=Nearest
  Triangle2 : simulink/Sources/Repeating Sequence  rep_seq_t=[0 1/fs/4 3/fs/4 1/fs]  rep_seq_y=[0 -1 1 0]
  Pulses : Outport
  wires:
  Mux/1 -> Pulses/1
  Relational Operator2/1 -> Mux/1, BL5/1
  BL5/1 -> Mux/2
  Relational Operator1/1 -> BL1/1, Mux/3
  Demux/1 -> Relational Operator2/2
  Triangle2/1 -> Relational Operator3/1, Relational Operator1/1, Relational Operator2/1
  BL1/1 -> Mux/4
  Relational Operator3/1 -> BL2/1, Mux/5
  BL2/1 -> Mux/6
  Demux/3 -> Relational Operator3/2
  Demux/2 -> Relational Operator1/2
  3Ph/1 -> Gain/1
  Gain/1 -> Demux/1

== matlab function parallel_battery_SC_boost_converter_new/MATLAB Function ==
  data: Vpv input; D output; Ipv input
function D = Pand0(Vpv, Ipv)

persistent Dprev Pprev Vprev

if isempty(Dprev)
    Dprev = 0.7;
    Vprev = 190;
    Pprev = 2000;
end

deltaD = 125e-6;

Ppv = Vpv*Ipv;

if (Ppv-Pprev) ~= 0
    if (Ppv-Pprev) > 0
        if (Vpv-Vprev) > 0
            D = Dprev - deltaD;
        else
            D = Dprev + deltaD;
        end
    else
        if (Vpv-Vprev) > 0
            D = Dprev + deltaD;
        else
            D = Dprev - deltaD;
        end
    end
else
    D = Dprev;
end


Dprev = D;
Vprev = Vpv;
Pprev = Ppv;
